simulink model "ABS_Structured_Bus"  (R2018a)
settings: Solver=ode45  StartTime=0  StopTime=10  FixedStep=0.001  RelTol=1e-3  AbsTol=1e-6
settings Model: ExtModeTrigMode=oneshot  ExtModeArmWhenConnect=off  Creator=ywata  LastModifiedBy=asun
settings SolverCC: AutoScaleAbsTol=off
settings DataIOCC: SaveFormat=Array  SignalLoggingSaveFormat=ModelDataLogs  SignalLoggingName=sigsOut
settings OptimizationCC: BlockReduction=off  BooleanDataType=off  LifeSpan=inf
settings DebuggingCC: SaveWithParameterizedLinksMsg=none  UnderspecifiedInitializationDetection=Classic  MergeDetectMultiDrivingBlocksExec=none  SignalResolutionControl=TryResolveAllWithWarning  MultiTaskDSMMsg=warning  MultiTaskCondExecSysMsg=none  FcnCallInpInsideContextMsg=warning  StateNameClashWarn=warning  SFUnexpectedBacktrackingDiag=warning  SFNoUnconditionalDefaultTransitionDiag=warning  SFExecutionAtInitializationDiag=none
settings HardwareCC: ProdBitPerPointer=32  ProdBitPerSizeT=32  ProdBitPerPtrDiffT=32  ProdLargestAtomicFloat=None  ProdIntDivRoundTo=Undefined  ProdEndianess=Unspecified  ProdWordSize=32  ProdHWDeviceType=32-bit Generic  TargetUnknown=on
settings ModelReferenceCC: EnableRefExpFcnMdlSchedulingChecks=off  PropagateSignalLabelsOutOfModel=off
settings RTWCC: TemplateMakefile=grt_vc.tmf
settings CodeAppCC: StateflowObjectComments=on
settings GRTTargetCC: TargetFcnLib=ansi_tfl_tmw.mat  TargetLangStandard=C89/C90 (ANSI)  CombineOutputUpdateFcns=off  GRTInterface=on
settings ConfigComp: CovMetricSettings=dw  CovSaveCumulativeToWorkspaceVar=on  CovSaveSingleToWorkspaceVar=on  CovExternalEMLEnable=off

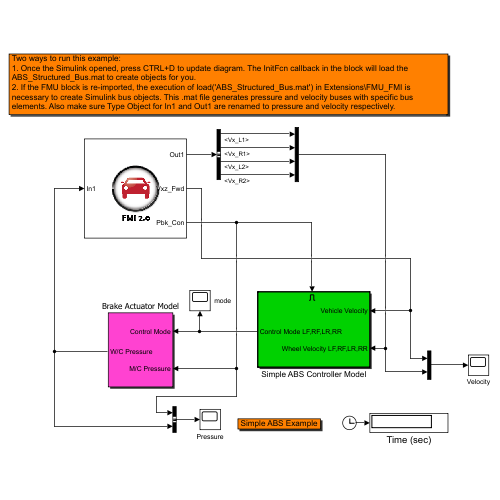
[thumbnail: Simulink's stored preview of the top-level diagram]
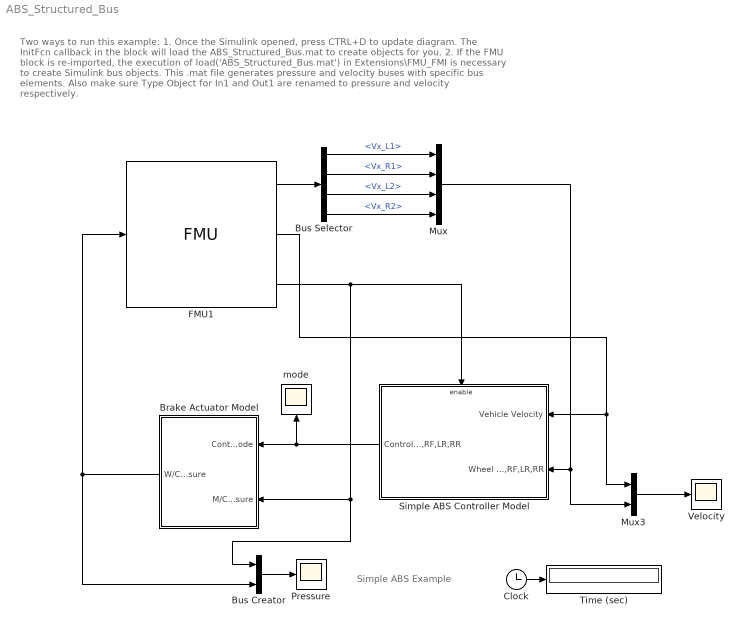
== system ABS_Structured_Bus ==
  note: Simple ABS Example
  note: Two ways to run this example:
      | 1. Once the Simulink opened, press CTRL+D to update diagram. The InitFcn callback in the block will load the ABS_Structured_Bus.mat to create objects for you.
      | 2. If the FMU block is re-imported, the execution of load('ABS_Structured_Bus.mat') in Extensions\FMU_FMI is necessary to create Simulink bus objects. This .mat file generates pressure and velocity buses with specific bus elements. Also make sure Type Object for In1 and Out1 are renamed to pressure and velocity respectively.
  Brake Actuator Model : Subsystem
  Bus Creator : BusCreator  Inputs=2
  Bus Selector : BusSelector  OutputSignals=Vx_L1,Vx_R1,Vx_L2,Vx_R2
  Clock : Clock
  FMU1 : FMU  InitFcn=load('ABS_Structured_Bus.mat')  FMUName=ABS_Structured_Bus.fmu  FMUMode=CoSimulation  FMUSampleTime=0.001
      mask Type: CarSim FMU -- FMI2.0 [Co-Simulation, v2.0]
      mask Display:
      | if (exist([Simulink.fileGenControl('get','CacheFolder') '\slprj\_fmu\3f0d5bfa88fc12597a5c9f6ca31c1c0e\ABS_Structured_Bus\model.png'],'file'))
      |     image([Simulink.fileGenControl('get','CacheFolder') '\slprj\_fmu\3f0d5bfa88fc12597a5c9f6ca31c1c0e\ABS_Structured_Bus\model.png']);
      | else
      |     disp('CarSim FMU -- FMI2.0');
      | end
      | port_label('output',1,'Out1');
      | port_label('output',2,'Vxz_Fwd');
      | port_label('output',3,'Pbk_Con');
      | port_label('input',1,'In1');
  Mux : Mux
  Mux3 : Mux  Inputs=2
  Pressure : Scope
  Simple ABS Controller Model : Subsystem
  Time (sec) : Display
      settings: Format=bank  Decimation=100
  Velocity : Scope
  mode : Scope
  wires:
  Bus Creator/1 -> Pressure/1
  FMU1/2 -> Mux3/1, Simple ABS Controller Model/1(Vehicle Velocity)
  Clock/1 -> Time (sec)/1
  Simple ABS Controller Model/1(Control Mode LF,RF,LR,RR) -> Brake Actuator Model/1(Control Mode), mode/1
  Brake Actuator Model/1(W/C Pressure) -> Bus Creator/2, FMU1/1
  Mux3/1 -> Velocity/1
  FMU1/3 -> Bus Creator/1, Brake Actuator Model/2(M/C Pressure), Simple ABS Controller Model/Enable
  Bus Selector/2 -> Mux/2  "<Vx_R1>"
  Bus Selector/1 -> Mux/1  "<Vx_L1>"
  FMU1/1 -> Bus Selector/1
  Mux/1 -> Mux3/2, Simple ABS Controller Model/2(Wheel Velocity LF,RF,LR,RR)
  Bus Selector/3 -> Mux/3  "<Vx_L2>"
  Bus Selector/4 -> Mux/4  "<Vx_R2>"

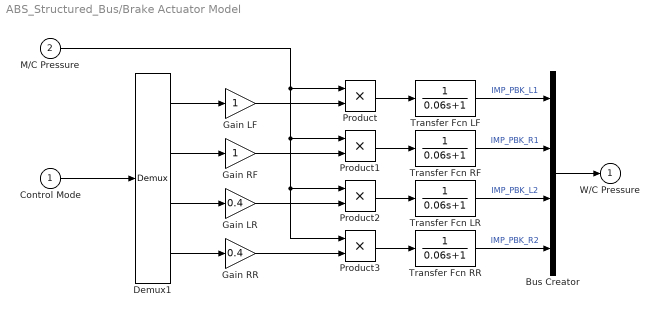
== system ABS_Structured_Bus/Brake Actuator Model ==
  Control Mode : Inport
  M/C Pressure : Inport  Port=2
  Bus Creator : BusCreator  Inputs=4  OutDataTypeStr=Bus: pressure  NonVirtualBus=on
  Demux1 : Demux
      settings: DisplayOption=none
  Gain LF : Gain  SaturateOnIntegerOverflow=on  OutDataTypeStr=Inherit: Same as input  ParamDataTypeStr=Inherit: Same as input
  Gain LR : Gain  Gain=0.4  SaturateOnIntegerOverflow=on  OutDataTypeStr=Inherit: Same as input  ParamDataTypeStr=Inherit: Same as input
  Gain RF : Gain  SaturateOnIntegerOverflow=on  OutDataTypeStr=Inherit: Same as input  ParamDataTypeStr=Inherit: Same as input
  Gain RR : Gain  Gain=0.4  SaturateOnIntegerOverflow=on  OutDataTypeStr=Inherit: Same as input  ParamDataTypeStr=Inherit: Same as input
  Product{,1..3} (4 alike) : Product  InputSameDT=on  SaturateOnIntegerOverflow=on  OutDataTypeStr=Inherit: Same as first input
  Transfer Fcn LF : TransferFcn  Denominator=[0.06 1]
  Transfer Fcn LR : TransferFcn  Denominator=[0.06 1]
  Transfer Fcn RF : TransferFcn  Denominator=[0.06 1]
  Transfer Fcn RR : TransferFcn  Denominator=[0.06 1]
  W/C Pressure : Outport  OutDataTypeStr=Bus: pressure  InitialOutput=0
  wires:
  Bus Creator/1 -> W/C Pressure/1
  Control Mode/1 -> Demux1/1
  Gain LF/1 -> Product/2
  Gain RF/1 -> Product1/2
  Gain LR/1 -> Product2/2
  Gain RR/1 -> Product3/2
  M/C Pressure/1 -> Product/1, Product1/1, Product2/1, Product3/1
  Product/1 -> Transfer Fcn LF/1
  Transfer Fcn LF/1 -> Bus Creator/1  "IMP_PBK_L1"
  Product1/1 -> Transfer Fcn RF/1
  Product2/1 -> Transfer Fcn LR/1
  Product3/1 -> Transfer Fcn RR/1
  Transfer Fcn LR/1 -> Bus Creator/3  "IMP_PBK_L2"
  Demux1/1 -> Gain LF/1
  Demux1/2 -> Gain RF/1
  Demux1/3 -> Gain LR/1
  Demux1/4 -> Gain RR/1
  Transfer Fcn RR/1 -> Bus Creator/4  "IMP_PBK_R2"
  Transfer Fcn RF/1 -> Bus Creator/2  "IMP_PBK_R1"

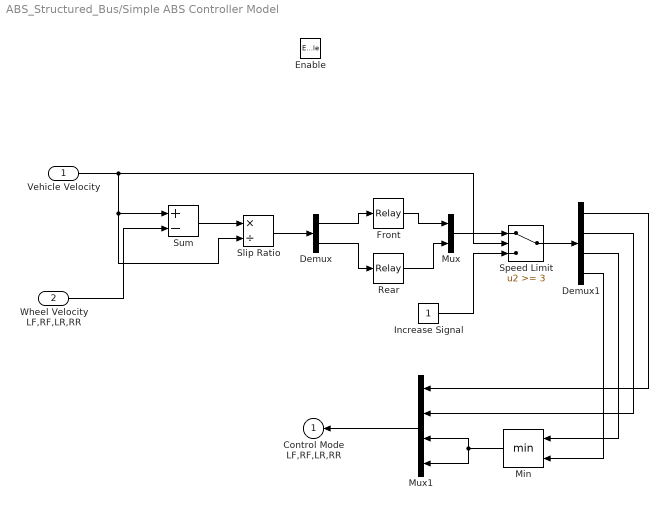
== system ABS_Structured_Bus/Simple ABS Controller Model ==
  Vehicle Velocity : Inport
  Wheel Velocity LF,RF,LR,RR : Inport  Port=2
  Enable : EnablePort
  Demux : Demux  Outputs=[2 2]
      settings: DisplayOption=none
  Demux1 : Demux
      settings: DisplayOption=none
  Front : Relay  OnSwitchValue=0.1  OffSwitchValue=0.05  OnOutputValue=0  OffOutputValue=1
  Increase Signal : Constant
  Min : MinMax  Inputs=2  InputSameDT=on  SaturateOnIntegerOverflow=on
  Mux : Mux  Inputs=2
  Mux1 : Mux
  Rear : Relay  OnSwitchValue=0.1  OffSwitchValue=0.05  OnOutputValue=0  OffOutputValue=1
  Slip Ratio : Product  Inputs=*/  InputSameDT=on  SaturateOnIntegerOverflow=on  OutDataTypeStr=Inherit: Same as first input
  Speed Limit : Switch  Threshold=3  SaturateOnIntegerOverflow=on  InputSameDT=on
  Sum : Sum  Inputs=+-  InputSameDT=on  SaturateOnIntegerOverflow=on  OutDataTypeStr=Inherit: Same as first input
  Control Mode LF,RF,LR,RR : Outport  InitialOutput=0
  wires:
  Vehicle Velocity/1 -> Sum/1, Slip Ratio/2, Speed Limit/2
  Speed Limit/1 -> Demux1/1
  Increase Signal/1 -> Speed Limit/3
  Sum/1 -> Slip Ratio/1
  Slip Ratio/1 -> Demux/1
  Mux/1 -> Speed Limit/1
  Min/1 -> Mux1/3, Mux1/4
  Demux1/3 -> Min/1
  Demux1/4 -> Min/2
  Demux1/2 -> Mux1/2
  Demux1/1 -> Mux1/1
  Mux1/1 -> Control Mode LF,RF,LR,RR/1
  Front/1 -> Mux/1
  Demux/1 -> Front/1
  Demux/2 -> Rear/1
  Rear/1 -> Mux/2
  Wheel Velocity LF,RF,LR,RR/1 -> Sum/2
